simulink model "om2"  (Simulink 7.2)
settings: Solver=ode45  StartTime=0.0  StopTime=10.0  RelTol=1e-3
libraries: cdsFilt x118, cdsEpicsOut x38, cdsIPC x23, cdsMatrix x10, cdsOsc x8, cdsPhaseDeg x8, cdsEpicsIn x8, cdsRms x8, cdsProduct x5, simulink x2, cdsWD x2, cdsIPCS x1
(part 4 of 6)

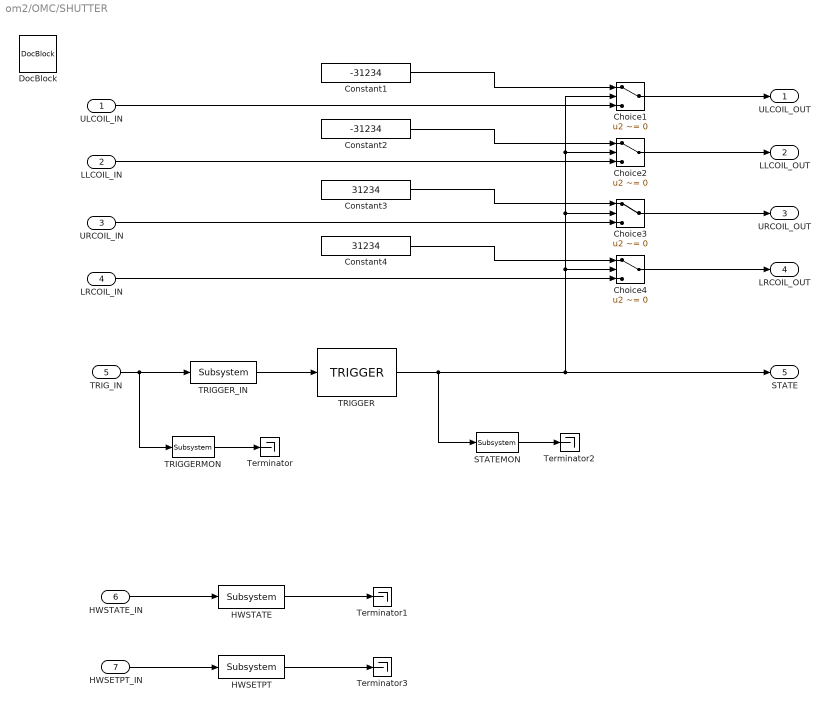
== system om2/OMC/SHUTTER ==
  ULCOIL_IN : Inport
  LLCOIL_IN : Inport  Port=2
  URCOIL_IN : Inport  Port=3
  LRCOIL_IN : Inport  Port=4
  TRIG_IN : Inport  Port=5
  HWSTATE_IN : Inport  Port=6
  HWSETPT_IN : Inport  Port=7
  Choice{1..4} (4 alike) : Switch  Criteria=u2 ~= 0
  Constant1 : Constant  Value=-31234  OutDataType=sfix(16)  OutScaling=2^0
  Constant2 : Constant  Value=-31234  OutDataType=sfix(16)  OutScaling=2^0
  Constant3 : Constant  Value=31234  OutDataType=sfix(16)  OutScaling=2^0
  Constant4 : Constant  Value=31234  OutDataType=sfix(16)  OutScaling=2^0
  DocBlock : simulink/Model-Wide Utilities/DocBlock  Tag=Overview  SystemSampleTime=-1  DocumentType=Text
      content=|
      | ---------------------------------------------------------------------------
      | OMC SHUTTER SUBSYSTEM
      | ---------------------------------------------------------------------------
      |
      | The designated parking position of the OMC tip-tilts is to divert the beam
      | downwards so that it hits the base of the OMC suspension.  Because the
      | magnets in the tip-tilts have differing polarities the signs of the
      | required actuation are not quite what you would expect.  Based on the
      | installed magnet configuration, the proper signal is:
      |
      | UL -
      | UR +
      | LR +
      | LL -
      |
      | Where those polarities are as seen in the VMON channels.
      |
      | Tobin Fricke <tfricke@ligo.caltech.edu>  May 3, 2008
      settings: AttributesFormatString=%<Tag>
  HWSETPT : cdsFilt/Subsystem  Tag=cdsFilt  Description=|  SystemSampleTime=-1
      | Purpose:                                                                                                                                                                                                                                  
      | Standard CDS IIR filter module.                                                                                                                                                                                                           
      |                                                                                                                                                                                                                                           
      | Operation:                                                                                                                                                                                                                                
      | Consists of 10 second order section IIR filters, plus a ramped gain stage. In FE code, also provides pre-defined test points and excitation channel inputs. The filter coefficients are defined in the LIGO system using the 'foton' tool.
      |                                                                                                                                                                                                                                           
      | Usage:                                                                                                                                                                                                                                    
      | Name the part with the desired filter module name.
      settings: AttributesFormatString=%<Tag>
  HWSTATE : cdsFilt/Subsystem  Tag=cdsFilt  Description=|  SystemSampleTime=-1
      | Purpose:                                                                                                                                                                                                                                  
      | Standard CDS IIR filter module.                                                                                                                                                                                                           
      |                                                                                                                                                                                                                                           
      | Operation:                                                                                                                                                                                                                                
      | Consists of 10 second order section IIR filters, plus a ramped gain stage. In FE code, also provides pre-defined test points and excitation channel inputs. The filter coefficients are defined in the LIGO system using the 'foton' tool.
      |                                                                                                                                                                                                                                           
      | Usage:                                                                                                                                                                                                                                    
      | Name the part with the desired filter module name.
      settings: AttributesFormatString=%<Tag>
  STATEMON : cdsEpicsOut/Subsystem  Tag=cdsEpicsOutput  Description=|  SystemSampleTime=-1
      | Purpose:                                          
      | Output a FE signal to an EPICS channel.           
      |                                                   
      | Operation:                                        
      | Takes input value and passes it to EPICS record.  
      |                                                   
      | Usage:                                            
      | Name the part with the desired EPICS rrecord name.
      settings: AttributesFormatString=%<Tag>
  TRIGGER : cdsTrigger/TRIGGER  Tag=cdsTrigger  SystemSampleTime=-1
      settings: AttributesFormatString=%<Tag>
  TRIGGERMON : cdsEpicsOut/Subsystem  Tag=cdsEpicsOutput  Description=|  SystemSampleTime=-1
      | Purpose:                                          
      | Output a FE signal to an EPICS channel.           
      |                                                   
      | Operation:                                        
      | Takes input value and passes it to EPICS record.  
      |                                                   
      | Usage:                                            
      | Name the part with the desired EPICS rrecord name.
      settings: AttributesFormatString=%<Tag>
  TRIGGER_IN : cdsFilt/Subsystem  Tag=cdsFilt  Description=|  SystemSampleTime=-1
      | Purpose:                                                                                                                                                                                                                                  
      | Standard CDS IIR filter module.                                                                                                                                                                                                           
      |                                                                                                                                                                                                                                           
      | Operation:                                                                                                                                                                                                                                
      | Consists of 10 second order section IIR filters, plus a ramped gain stage. In FE code, also provides pre-defined test points and excitation channel inputs. The filter coefficients are defined in the LIGO system using the 'foton' tool.
      |                                                                                                                                                                                                                                           
      | Usage:                                                                                                                                                                                                                                    
      | Name the part with the desired filter module name.
      settings: AttributesFormatString=%<Tag>
  Terminator{,1..3} (4 alike) : Terminator
  ULCOIL_OUT : Outport
  LLCOIL_OUT : Outport  Port=2
  URCOIL_OUT : Outport  Port=3
  LRCOIL_OUT : Outport  Port=4
  STATE : Outport  Port=5
  wires:
  TRIG_IN/1 -> TRIGGERMON/1, TRIGGER_IN/1
  TRIGGERMON/1 -> Terminator/1
  STATEMON/1 -> Terminator2/1
  Choice1/1 -> ULCOIL_OUT/1
  Choice2/1 -> LLCOIL_OUT/1
  Choice3/1 -> URCOIL_OUT/1
  Choice4/1 -> LRCOIL_OUT/1
  TRIGGER/1 -> STATEMON/1, STATE/1, Choice1/2, Choice2/2, Choice3/2, Choice4/2
  HWSTATE_IN/1 -> HWSTATE/1
  HWSETPT_IN/1 -> HWSETPT/1
  HWSTATE/1 -> Terminator1/1
  HWSETPT/1 -> Terminator3/1
  TRIGGER_IN/1 -> TRIGGER/1
  Constant1/1 -> Choice1/1
  Constant2/1 -> Choice2/1
  Constant3/1 -> Choice3/1
  Constant4/1 -> Choice4/1
  ULCOIL_IN/1 -> Choice1/3
  LLCOIL_IN/1 -> Choice2/3
  URCOIL_IN/1 -> Choice3/3
  LRCOIL_IN/1 -> Choice4/3
